simulink model "motion_robot"  (Simulink 10.0)
settings: Solver=FixedStepAuto  StartTime=0.0  StopTime=60  FixedStep=fixedStep  MaxStep=0.2  RelTol=1e-3
values from neighbouring files (symbols this model uses):
  sensitivityDis = 1    [motionSensorInit.m]
undefined symbols (not defined in the file or in its folder): robotDis, startRobot, timeRobot
settings Model: Creator=lixuansong  LastModifiedBy=lixuansong
settings DataIOCC: SaveFormat=Dataset  ReturnWorkspaceOutputs=on
settings OptimizationCC: LifeSpan=auto
settings DebuggingCC: UnderspecifiedInitializationDetection=Simplified  MergeDetectMultiDrivingBlocksExec=error  SFUnexpectedBacktrackingDiag=error  SFNoUnconditionalDefaultTransitionDiag=error  SFExecutionAtInitializationDiag=warning  ArithmeticOperatorsInVariantConditions=error
settings HardwareCC: ProdBitPerPointer=64  ProdBitPerSizeT=64  ProdBitPerPtrDiffT=64  ProdLargestAtomicFloat=Float  ProdIntDivRoundTo=Zero  ProdEndianess=LittleEndian  ProdWordSize=64  ProdHWDeviceType=Intel->x86-64 (Windows64)
settings ModelReferenceCC: PropagateSignalLabelsOutOfModel=on
settings SFSimCC: SimUseLocalCustomCode=on  CustomCodeUndefinedFunction=FilterOut
settings RTWCC: RTWUseLocalCustomCode=on
settings CodeAppCC: StateflowObjectComments=off
settings GRTTargetCC: TargetLangStandard=C99 (ISO)  CombineOutputUpdateFcns=on  GRTInterface=off
settings ConfigComp: CovMetricSettings=dwe  CovHtmlReporting=off  CovSaveCumulativeToWorkspaceVar=off  CovSaveSingleToWorkspaceVar=off

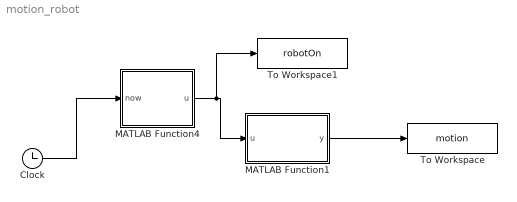
== system motion_robot ==
  Clock : Clock
  MATLAB Function1 : MATLAB Function  TreatAsAtomicUnit=on
  MATLAB Function4 : MATLAB Function  TreatAsAtomicUnit=on
  To Workspace : ToWorkspace  VariableName=motion  SampleTime=-1
  To Workspace1 : ToWorkspace  VariableName=robotOn  SampleTime=-1
  wires:
  MATLAB Function4/1(u) -> MATLAB Function1/1(u), To Workspace1/1
  Clock/1 -> MATLAB Function4/1(now)
  MATLAB Function1/1(y) -> To Workspace/1

== matlab function MATLAB Function1 ==
  data: u input double; y output double; sensitivityDis parameter double; robotDis parameter double
function y = motionDetector(u,sensitivityDis, robotDis)

if robotDis<=sensitivityDis
    y=u;
else
    y=0;
end

== matlab function MATLAB Function4 ==
  data: u output double; now input double; startRobot parameter double; timeRobot parameter double
function u = controlRobot(now,startRobot,timeRobot)
if now>=startRobot && now<=startRobot+timeRobot
    u=1;
else
    u=0;
end
